simulink model "Child_Phone"  (R2023a)
settings: Solver=FixedStepDiscrete  StartTime=0.0  StopTime=100  RelTol=1e-3
undefined symbols (not defined in the file): Child_Safety, Lat
libraries: androidcommunicationlib x9, androidsensorlib x5, androidaudiovideolib x4, androiduilib x3
settings Model: Creator=91940  LastModifiedBy=dhart
settings OptimizationCC: EnhancedBackFolding=on  PassReuseOutputArgsAs=Individual arguments  ZeroExternalMemoryAtStartup=off  ZeroInternalMemoryAtStartup=off  MaxStackSize=64  OptimizeBlockOrder=speed  DifferentSizesBufferReuse=on  OptimizationCustomize=off  EfficientTunableParamExpr=on
settings DebuggingCC: ParameterTunabilityLossMsg=error
settings HardwareCC: ProdBitPerPointer=32  ProdBitPerSizeT=32  ProdBitPerPtrDiffT=32  ProdLargestAtomicInteger=Long  ProdLargestAtomicFloat=Double  ProdWordSize=32  ProdHWDeviceType=ARM Compatible->ARM Cortex
settings ModelReferenceCC: EnableRefExpFcnMdlSchedulingChecks=on
settings SFSimCC: MATLABDynamicMemAlloc=off
settings RTWCC: Description=Embedded Coder  SystemTargetFile=ert.tlc  HardwareBoard=Android Device  TLCOptions="-aInlineSetEventsForThisBaseRateFcn=TLC_FALSE -aSuppressMultiTaskScheduler=TLC_FALSE  -aRateBasedStepFcn=0"  TemplateMakefile=ert_default_tmf  RTWVerbose=off  Toolchain=Android SDK/NDK Tools  BuildConfiguration=Faster Runs
settings CodeAppCC: ForceParamTrailComments=on  IgnoreCustomStorageClasses=off  OperatorAnnotations=on  SimulinkDataObjDesc=on  SFDataObjDesc=on  InsertBlockDesc=on

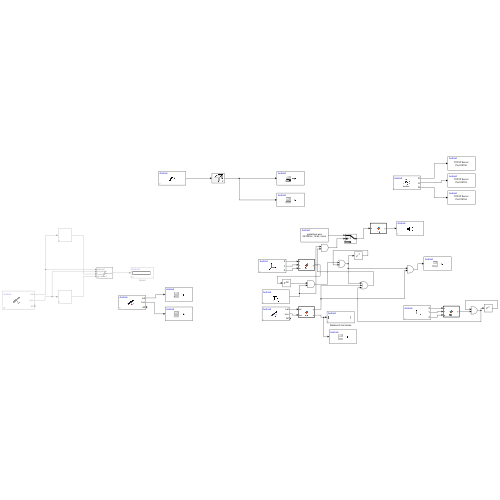
[thumbnail: Simulink's stored preview of the top-level diagram]
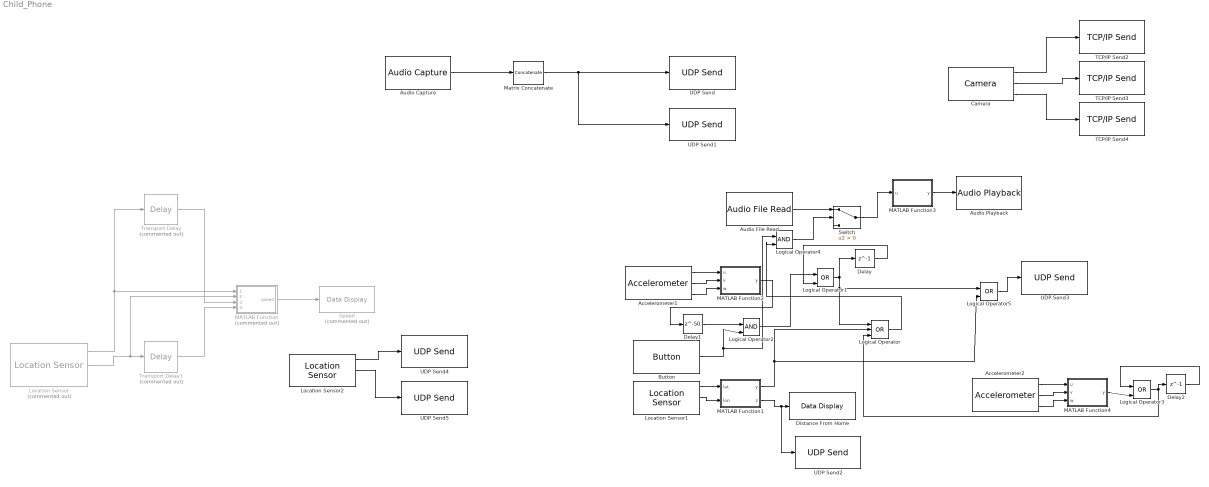
== system Child_Phone ==
  Accelerometer1 : androidsensorlib/Accelerometer  OutputVector=off  SampleTime=0.1  BlockPlatform=Android
  Accelerometer2 : androidsensorlib/Accelerometer  OutputVector=off  SampleTime=0.1  BlockPlatform=Android
  Audio Capture : androidaudiovideolib/Audio Capture  SampleFreq=44100  FrameSize=4410  SampleTime=0.1  SimulateUsing=Code generation  DeviceStr=0  QueueDuration=0  BlockPlatform=Android  AudioSamplingFreq=44100
  Audio File Read : androidaudiovideolib/Audio File Read  FileName=C:\Users\91940\Downloads\beep-01a.wav  FrameSize=4410
  Audio Playback : androidaudiovideolib/Audio Playback  SampleFreq=44100  AudioSamplingFreq=44100  SampleTime=0.1  DeviceStr=0  QueueDuration=0  BlockPlatform=Android
  Button : androiduilib/Button  ButtonState=Pressed  ButtonId=Child_Phone/Button  State=on  SampleTime=0.1  BlockPlatform=Android
  Camera : androidaudiovideolib/Camera  CameraLocation=Back  CameraResolutions=Back - 640x480  Width=640  Height=480  SampleTime=2  BlockPlatform=Android
  Delay : Delay  DelayLength=1  InitialCondition=0
  Delay1 : Delay  DelayLength=50  InitialCondition=0
  Delay2 : Delay  DelayLength=1  InitialCondition=0
  Distance From Home : androiduilib/Data Display  DataDisplayId=Child_Phone/Distance_From_Home  Format=Float  Precision=6  SimulateUsing=Code generation  blockPlatform=Android
  Location Sensor : androidsensorlib/Location Sensor  Commented=on  OutputVector=off  SampleTime=0.1  BlockPlatform=Android
  Location Sensor1 : androidsensorlib/Location Sensor  OutputVector=off  SampleTime=0.1  BlockPlatform=Android
  Location Sensor2 : androidsensorlib/Location Sensor  OutputVector=off  SampleTime=0.1  BlockPlatform=Android
  Logical Operator : Logic  Operator=OR  Inputs=3  IconShape=distinctive  AllPortsSameDT=off  OutDataTypeStr=boolean
  Logical Operator1 : Logic  Operator=OR  IconShape=distinctive  AllPortsSameDT=off  OutDataTypeStr=boolean
  Logical Operator2 : Logic  IconShape=distinctive  AllPortsSameDT=off  OutDataTypeStr=boolean
  Logical Operator3 : Logic  Operator=OR  IconShape=distinctive  AllPortsSameDT=off  OutDataTypeStr=boolean
  Logical Operator4 : Logic  IconShape=distinctive  AllPortsSameDT=off  OutDataTypeStr=boolean
  Logical Operator5 : Logic  Operator=OR  IconShape=distinctive  AllPortsSameDT=off  OutDataTypeStr=boolean
  MATLAB Function : MATLAB Function  Commented=on  TreatAsAtomicUnit=on
  MATLAB Function1 : MATLAB Function  TreatAsAtomicUnit=on
  MATLAB Function2 : MATLAB Function  TreatAsAtomicUnit=on
  MATLAB Function3 : MATLAB Function  TreatAsAtomicUnit=on
  MATLAB Function4 : MATLAB Function  TreatAsAtomicUnit=on
  Matrix Concatenate : Concatenate  NumInputs=1  Mode=Multidimensional array  ConcatenateDimension=2
  Speed : androiduilib/Data Display  Commented=on  DataDisplayId=Child_Safety/Lat  Format=Float  Precision=6  SimulateUsing=Code generation  blockPlatform=Android
  Switch : Switch  Criteria=u2 > Threshold  SaturateOnIntegerOverflow=off  InputSameDT=off
  TCP/IP Send2 : androidcommunicationlib/TCP//IP Send  TCPSendId=Child_Phone/TCP//IP_Send2  Mode_=Server  LocalServerPort_=39152  RemoteAddr_=127.0.0.1  RemoteServerPort_=25152  ClientPortBindingSelection_=off  ClientPortToBind_=35000  BlockingMode_=off  BlockTimeout_=0.1
  TCP/IP Send3 : androidcommunicationlib/TCP//IP Send  TCPSendId=Child_Phone/TCP//IP_Send3  Mode_=Server  LocalServerPort_=39153  RemoteAddr_=127.0.0.1  RemoteServerPort_=25152  ClientPortBindingSelection_=off  ClientPortToBind_=35000  BlockingMode_=off  BlockTimeout_=0.1
  TCP/IP Send4 : androidcommunicationlib/TCP//IP Send  TCPSendId=Child_Phone/TCP//IP_Send4  Mode_=Server  LocalServerPort_=39154  RemoteAddr_=127.0.0.1  RemoteServerPort_=25152  ClientPortBindingSelection_=off  ClientPortToBind_=35000  BlockingMode_=off  BlockTimeout_=0.1
  Transport Delay : TransportDelay  Commented=on  DelayTime=2
  Transport Delay1 : TransportDelay  Commented=on  DelayTime=2
  UDP Send : androidcommunicationlib/UDP Send  remoteURL='10.7.9.90'  remotePort=39155  localURL='0.0.0.0'  localPortSource=Automatically determine  localPort=-1  sampletime=-1  blockPlatform=Android  separateLengthPort=0
  UDP Send1 : androidcommunicationlib/UDP Send  remoteURL='10.7.9.90'  remotePort=39156  localURL='0.0.0.0'  localPortSource=Automatically determine  localPort=-1  sampletime=-1  blockPlatform=Android  separateLengthPort=0
  UDP Send2 : androidcommunicationlib/UDP Send  remoteURL='10.7.9.90'  remotePort=39150  localURL='0.0.0.0'  localPortSource=Automatically determine  localPort=-1  sampletime=-1  blockPlatform=Android  separateLengthPort=0
  UDP Send3 : androidcommunicationlib/UDP Send  remoteURL='10.7.9.90'  remotePort=39157  localURL='0.0.0.0'  localPortSource=Automatically determine  localPort=-1  sampletime=-1  blockPlatform=Android  separateLengthPort=0
  UDP Send4 : androidcommunicationlib/UDP Send  remoteURL='10.7.9.90'  remotePort=39158  localURL='0.0.0.0'  localPortSource=Automatically determine  localPort=-1  sampletime=-1  blockPlatform=Android  separateLengthPort=0
  UDP Send5 : androidcommunicationlib/UDP Send  remoteURL='10.7.9.90'  remotePort=39159  localURL='0.0.0.0'  localPortSource=Automatically determine  localPort=-1  sampletime=-1  blockPlatform=Android  separateLengthPort=0
  wires:
  Location Sensor/1 -> Transport Delay/1, MATLAB Function/1(latitude1)
  Location Sensor/2 -> MATLAB Function/2(longitude1), Transport Delay1/1
  Transport Delay/1 -> MATLAB Function/3(latitude2)
  Transport Delay1/1 -> MATLAB Function/4(longitude2)
  MATLAB Function/1(speed) -> Speed/1
  Location Sensor1/1 -> MATLAB Function1/1(lat)
  Location Sensor1/2 -> MATLAB Function1/2(lon)
  MATLAB Function1/2(z) -> UDP Send2/1, Distance From Home/1
  MATLAB Function1/1(y) -> Logical Operator/2, Logical Operator5/2
  Accelerometer1/1 -> MATLAB Function2/1(u)
  Accelerometer1/2 -> MATLAB Function2/2(v)
  Accelerometer1/3 -> MATLAB Function2/3(w)
  Logical Operator1/1 -> Logical Operator5/1, Logical Operator/1, Delay/1
  Delay/1 -> Logical Operator1/2
  Audio File Read/1 -> Switch/1
  Switch/1 -> MATLAB Function3/1(u)
  MATLAB Function3/1(y) -> Audio Playback/1
  Audio Capture/1 -> Matrix Concatenate/1
  Matrix Concatenate/1 -> UDP Send1/1, UDP Send/1
  Camera/1 -> TCP/IP Send2/1
  Camera/2 -> TCP/IP Send3/1
  Camera/3 -> TCP/IP Send4/1
  MATLAB Function2/1(y) -> Delay1/1
  Button/1 -> Logical Operator4/1, Logical Operator2/2
  Delay1/1 -> Logical Operator2/1
  Location Sensor2/1 -> UDP Send4/1
  Location Sensor2/2 -> UDP Send5/1
  Logical Operator2/1 -> Logical Operator1/1
  Accelerometer2/2 -> MATLAB Function4/2(v)
  Delay2/1 -> Logical Operator3/1
  Accelerometer2/3 -> MATLAB Function4/3(w)
  Logical Operator3/1 -> Delay2/1, Logical Operator/3
  Accelerometer2/1 -> MATLAB Function4/1(u)
  MATLAB Function4/1(y) -> Logical Operator3/2
  Logical Operator/1 -> Logical Operator4/2
  Logical Operator4/1 -> Switch/2
  Logical Operator5/1 -> UDP Send3/1

== matlab function Child_Phone/MATLAB Function1 ==
  data: lat input; y output; lon input; z output
function [y,z]= fcn(lat, lon)
 % Haversine formula to calculate distance between two points on Earth
    R = 6371; % Earth's radius in kilometers
    radius = 0.1;
    lat1_rad = deg2rad(23.210406);
    lon1_rad = deg2rad(72.683669);
    lat2_rad = deg2rad(lat);
    lon2_rad = deg2rad(lon);
    dlat = lat2_rad - lat1_rad;
    dlon = lon2_rad - lon1_rad;
    a = sin(dlat/2)^2 + cos(lat1_rad) * cos(lat2_rad) * sin(dlon/2)^2;
    c = 2 * atan2(sqrt(a), sqrt(1-a));
    distance = R * c;
    z = distance;
    
    % Check if the distance is greater than the specified radius
    if distance > radius
        y = 1; % Point is outside the specified radius
    else
        y = 0; % Point is inside or on the specified radius
    end
end

== matlab function Child_Phone/MATLAB Function ==
  data: latitude1 input; speed output; longitude1 input; latitude2 input; longitude2 input

    function speed = fcn(latitude1, longitude1, latitude2, longitude2)
    % Earth radius (in kilometers)
    R = 6371;

    % Convert latitude and longitude from degrees to radians
    lat1 = deg2rad(latitude1);
    lon1 = deg2rad(longitude1);
    lat2 = deg2rad(latitude2);
    lon2 = deg2rad(longitude2);

    % Haversine formula to calculate distance
    deltaLat = lat2 - lat1;
    deltaLon = lon2 - lon1;
    a = sin(deltaLat/2)^2 + cos(lat1) * cos(lat2) * sin(deltaLon/2)^2;
    c = 2 * atan2(sqrt(a), sqrt(1-a));
    distance = R * c;

    % Calculate speed
    speed = distance /2;
end

== matlab function Child_Phone/MATLAB Function2 ==
  data: u input; y output; v input; w input
function y = fcn(u, v, w)
    if (u^2 + v^2 + w^2)^(1/2) > 50
        y =1;
    else
        y=0;
    end
end

== matlab function Child_Phone/MATLAB Function3 ==
  data: u input; y output
function y = fcn(u)
    y = [u,u];
end

== matlab function Child_Phone/MATLAB Function4 ==
  data: u input; y output; v input; w input
function y = fcn(u, v, w)
    if (u^2 + v^2 + w^2)^(1/2) > 50
        y =1;
    else
        y=0;
    end
end
